simulink model "PID_clasic"  (R2022a)
settings: Solver=VariableStepAuto  StartTime=0.0  StopTime=100  RelTol=1e-3
values from neighbouring files (symbols this model uses):
  A1 = [1 -0.297456502745 0.0957579468989 -0.192633039978 -0.0987226489635 -0.0728334914316 -0.156676215523 0.0775890223397 -0.0843119777096 0.0177077980777 -0.195182528996 0.00108869630591 ... (31 elements, 1x31)]    [ASTANK2_date_model.mat]    (also in workspace_final.mat)
  A2 = [1 -0.270802539442 0.170850582191 -0.229570308505 0.0102319327613 -0.18532557909 -0.113714973821 -0.153704056044 -0.0527641928514 -0.128387187818 -0.0711693493773 -0.0510682923372 ... (28 elements, 1x28)]    [ASTANK2_date_model.mat]    (also in workspace_final.mat)
  B11 = [0 0.00944944705063 0.0281682614784 0.0334217172474 -0.0139674115853 0.0118573023308 -0.0458082800907 0.0127541748473 -0.0229098962043 0.0376416216646 -0.0113334758876 0.0501709318659 ... (23 elements, 1x23)]    [ASTANK2_date_model.mat]    (also in workspace_final.mat)
  B12 = [0 -0.0371516935398 0.0070714627159 0.00750897045034 -0.0357970892593 0.00682665229691 0.000906798594331 0.036803959743 -0.0164721886728 0.0137196915339 0.000966304479888 -0.0420499575352 ... (17 elements, 1x17)]    [ASTANK2_date_model.mat]    (also in workspace_final.mat)
  B21 = [0 0.00483083228197 -0.0385678930745 0.0353410298705 0.000889493008077 -0.119047801697 0.053906249607 0.0692127962007]    [ASTANK2_date_model.mat]    (also in workspace_final.mat)
  B22 = [0 0.0558812162712 -0.0416154850143 0.0764500077791 0.0184452097899 0.0332231193511 -0.0329558124428 0.0133387456409 -0.0103666234705 0.0473107779539 -0.00799935838997 -0.00686596320156 ... (27 elements, 1x27)]    [ASTANK2_date_model.mat]    (also in workspace_final.mat)
  C1 = [1 0.27606315627 -0.0342575988634 0.134269396132 0.194125022115 0.112736561519 0.201227895715 0.0732341463885 0.137846883145 0.144137916166 0.306934687093 0.162394775686 ... (66 elements, 1x66)]    [ASTANK2_date_model.mat]    (also in workspace_final.mat)
  C2 = [1 0.289146669342 -0.069344975204 0.169786493921 0.132040170853 0.177089391805 0.208658182826 0.19392989144 0.211932940321 0.217587694817 0.25271491779 0.248422499665 ... (96 elements, 1x96)]    [ASTANK2_date_model.mat]    (also in workspace_final.mat)
  D1 = 1    [ASTANK2_date_model.mat]    (also in workspace_final.mat)
  D2 = 1    [ASTANK2_date_model.mat]    (also in workspace_final.mat)
  Kp_z = [Kp_11 Kp_12; Kp_21 Kp_22]    [PSO.m]    (also in PSO_init.m; PSO_initD.m; evaluatePID.m; workspace_final.mat = [1  0.103038272484; 0.750995048664  0.878106954466])
libraries: simulink x2, cstblocks x2
settings Model: Creator=Dragos  LastModifiedBy=drago
settings ModelReferenceCC: EnableRefExpFcnMdlSchedulingChecks=off
settings RTWCC: Description=Generic Real-Time Target  GPUComputeCapability=5.0

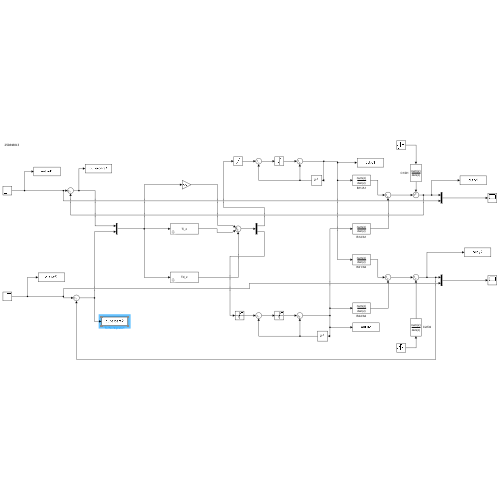
[thumbnail: Simulink's stored preview of the top-level diagram]
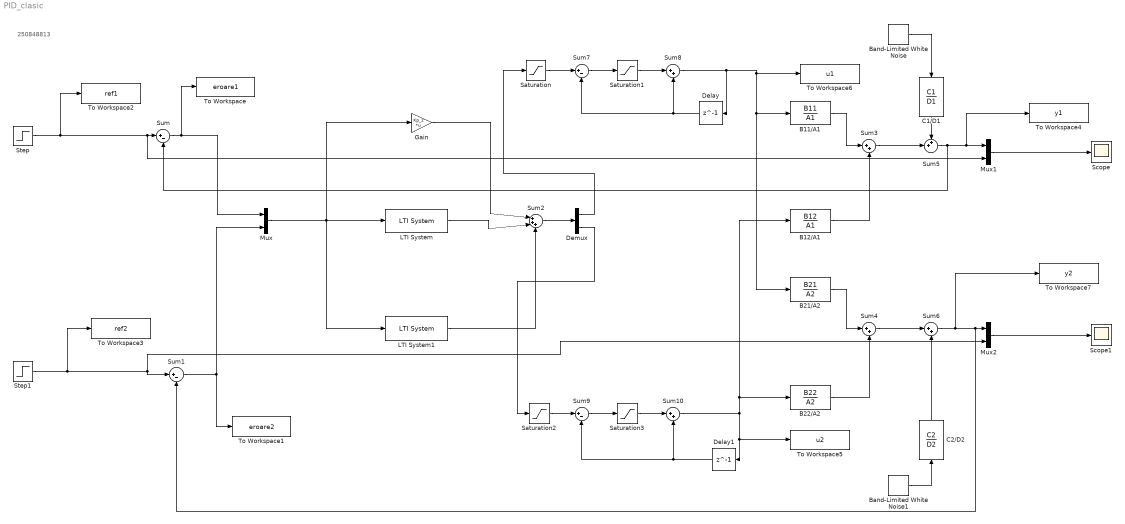
== system PID_clasic ==
  note: 250848813
  B11/A1 : DiscreteFilter  Numerator=B11  Denominator=A1
  B12/A1 : DiscreteFilter  Numerator=B12  Denominator=A1
  B21/A2 : DiscreteFilter  Numerator=B21  Denominator=A2
  B22/A2 : DiscreteFilter  Numerator=B22  Denominator=A2
  Band-Limited White Noise : simulink/Sources/Band-Limited White Noise  Cov=lambda1  Ts=1  seed=[23341]
  Band-Limited White Noise1 : simulink/Sources/Band-Limited White Noise  Cov=lambda2  Ts=1  seed=[23341]
  C1/D1 : DiscreteFilter  Numerator=C1  Denominator=D1
  C2/D2 : DiscreteFilter  Numerator=C2  Denominator=D2
  Delay : Delay  DelayLength=1
  Delay1 : Delay  DelayLength=1
  Demux : Demux  Outputs=2
  Gain : Gain  Gain=Kp_z  Multiplication=Matrix(K*u)
  LTI System : cstblocks/LTI System  sys=Ti_z  IC=[]
  LTI System1 : cstblocks/LTI System  sys=Td_z  IC=[]
  Mux : Mux  Inputs=2
  Mux1 : Mux  Inputs=2
  Mux2 : Mux  Inputs=2
  Saturation : Saturate  UpperLimit=10  LowerLimit=2
  Saturation1 : Saturate  UpperLimit=3  LowerLimit=-3
  Saturation2 : Saturate  UpperLimit=10  LowerLimit=2
  Saturation3 : Saturate  UpperLimit=3  LowerLimit=-3
  Scope : Scope
  Scope1 : Scope
  Step : Step  Time=0  After=9  SampleTime=0
  Step1 : Step  Time=0  After=10  SampleTime=0
  Sum{,1,7,9} (4 alike) : Sum  Inputs=|+-
  Sum{3..4,6,8,10} (5 alike) : Sum  Inputs=|++
  Sum2 : Sum  Inputs=|+++
  Sum5 : Sum  Inputs=++|
  To Workspace : ToWorkspace  VariableName=eroare1  SampleTime=1
      settings: Save2DSignal=2-D array (concatenate along first dimension)
  To Workspace1 : ToWorkspace  VariableName=eroare2  SampleTime=1
      settings: Save2DSignal=2-D array (concatenate along first dimension)
  To Workspace2 : ToWorkspace  VariableName=ref1  SampleTime=1
      settings: Save2DSignal=2-D array (concatenate along first dimension)
  To Workspace3 : ToWorkspace  VariableName=ref2  SampleTime=1
      settings: Save2DSignal=2-D array (concatenate along first dimension)
  To Workspace4 : ToWorkspace  VariableName=y1  SampleTime=1
      settings: Save2DSignal=2-D array (concatenate along first dimension)
  To Workspace5 : ToWorkspace  VariableName=u2  SampleTime=1
      settings: Save2DSignal=2-D array (concatenate along first dimension)
  To Workspace6 : ToWorkspace  VariableName=u1  SampleTime=1
      settings: Save2DSignal=2-D array (concatenate along first dimension)
  To Workspace7 : ToWorkspace  VariableName=y2  SampleTime=1
      settings: Save2DSignal=2-D array (concatenate along first dimension)
  wires:
  Step/1 -> To Workspace2/1, Mux1/2, Sum/1
  Step1/1 -> To Workspace3/1, Sum1/1, Mux2/2
  Sum/1 -> To Workspace/1, Mux/1
  Sum1/1 -> To Workspace1/1, Mux/2
  Mux/1 -> LTI System/1, Gain/1, LTI System1/1
  Gain/1 -> Sum2/1
  Sum2/1 -> Demux/1
  B11/A1/1 -> Sum3/1
  B12/A1/1 -> Sum3/2
  B21/A2/1 -> Sum4/1
  B22/A2/1 -> Sum4/2
  C1/D1/1 -> Sum5/1
  Sum3/1 -> Sum5/2
  Sum4/1 -> Sum6/1
  C2/D2/1 -> Sum6/2
  Sum5/1 -> Sum/2, To Workspace4/1, Mux1/1
  Mux1/1 -> Scope/1
  Sum6/1 -> To Workspace7/1, Sum1/2, Mux2/1
  Mux2/1 -> Scope1/1
  Band-Limited White Noise/1 -> C1/D1/1
  Band-Limited White Noise1/1 -> C2/D2/1
  LTI System1/1 -> Sum2/3
  LTI System/1 -> Sum2/2
  Saturation/1 -> Sum7/1
  Sum7/1 -> Saturation1/1
  Saturation1/1 -> Sum8/1
  Delay/1 -> Sum7/2, Sum8/2
  Sum8/1 -> Delay/1, B21/A2/1, B11/A1/1, To Workspace6/1
  Demux/1 -> Saturation/1
  Saturation2/1 -> Sum9/1
  Sum9/1 -> Saturation3/1
  Saturation3/1 -> Sum10/1
  Delay1/1 -> Sum9/2, Sum10/2
  Sum10/1 -> To Workspace5/1, Delay1/1, B22/A2/1, B12/A1/1
  Demux/2 -> Saturation2/1
